simulink library "EPSI_lib"  (Simulink 7.5)
settings: Solver=ode45  StartTime=0.0  StopTime=10.0  RelTol=1e-3
libraries: PES_CZ_FAW x1, simulink x1
settings Model: Creator=wuaibin  LastModifiedBy=wuaibin

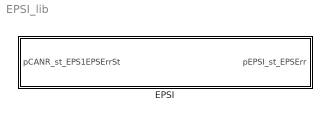
== system EPSI_lib ==
  EPSI : Subsystem  TreatAsAtomicUnit=on

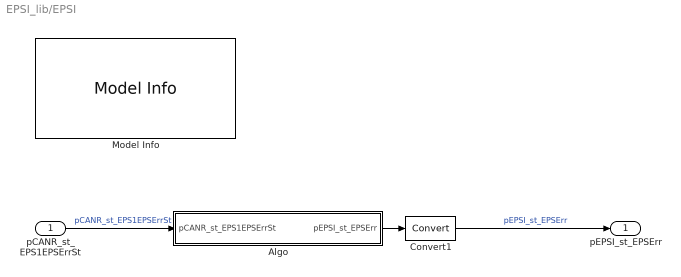
== system EPSI_lib/EPSI ==
  pCANR_st_EPS1EPSErrSt : Inport  OutDataType=fixdt(1, 16)  OutScaling=2^0
  Algo : Subsystem
  Convert1 : DataTypeConversion  OutDataType=fixdt(1, 16)  OutScaling=2^0
  Model Info : simulink/Model-Wide Utilities/Model Info  SystemSampleTime=-1  InitialBlockCM=None  BlockCM=None  Frame=on  DisplayStringWithTags=Model Info\nCreated: %<Created>\nCreator: %<Creator>  HorizontalTextAlignment=Center  LeftAlignmentValue=0.5  SourceBlockDiagram=HQEV_HCU  TagMaxNumber=20
  pEPSI_st_EPSErr : Outport  OutDataType=fixdt(1, 16)  OutScaling=2^0
  wires:
  Convert1/1 -> pEPSI_st_EPSErr/1  "pEPSI_st_EPSErr"
  Algo/1(pEPSI_st_EPSErr) -> Convert1/1
  pCANR_st_EPS1EPSErrSt/1 -> Algo/1(pCANR_st_EPS1EPSErrSt)  "pCANR_st_EPS1EPSErrSt"

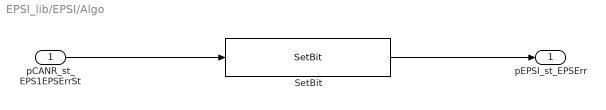
== system EPSI_lib/EPSI/Algo ==
  pCANR_st_EPS1EPSErrSt : Inport  OutDataType=fixdt(1, 16)  OutScaling=2^0
  SetBit : PES_CZ_FAW/Discontinuities/SetBit  SystemSampleTime=-1  maska=FAWEpsErrTyp.EPS_ERROR
  pEPSI_st_EPSErr : Outport  OutDataType=fixdt(1, 16)  OutScaling=2^0
  wires:
  SetBit/1 -> pEPSI_st_EPSErr/1
  pCANR_st_EPS1EPSErrSt/1 -> SetBit/1
